simulink model "RiceCooker_harness0"  (R2023b)
settings: Solver=VariableStepAuto  StartTime=0.0  StopTime=5  RelTol=1e-3
settings Model: Creator=20181234  LastModifiedBy=20181234

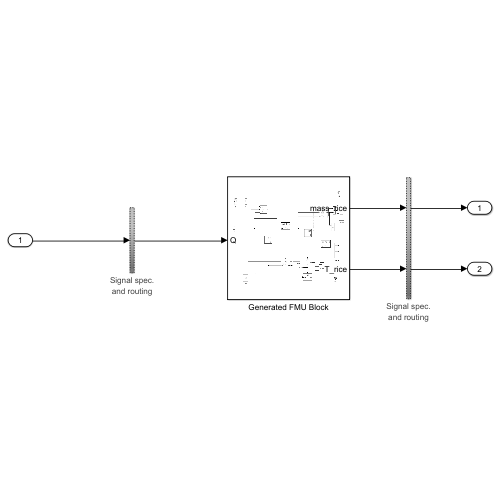
[thumbnail: Simulink's stored preview of the top-level diagram]
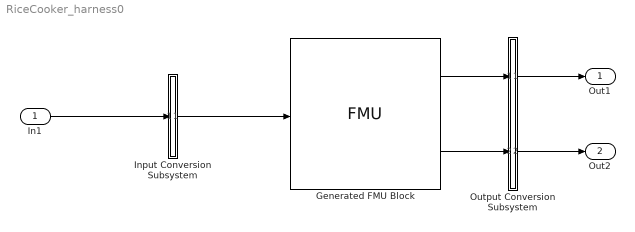
== system RiceCooker_harness0 ==
  In1 : Inport  OutDataTypeStr=double  PortDimensions=[1]  SampleTime=1
  Generated FMU Block : FMU  FMUName=RiceCooker  FMUMode=CoSimulation  FMUSampleTime=1  FMUCreateBusObject=off  FMUInitializeEnumObject=off  T_0=100  m_0=1.5  mask(RiceCooker [Co-Simulation, v2.0]){}
      mask Display:
      | if (exist([Simulink.fileGenControl('get','CacheFolder') '\slprj\_fmu\fd06c610bd597baabc11c1582149db8f\RiceCooker\model.png'],'file'))
      |     image([Simulink.fileGenControl('get','CacheFolder') '\slprj\_fmu\fd06c610bd597baabc11c1582149db8f\RiceCooker\model.png']);
      | else
      |     disp('RiceCooker');
      | end
      | port_label('output',1,'mass_rice');
      | port_label('output',2,'T_rice');
      | port_label('input',1,'Q');
  Input Conversion Subsystem : Subsystem  Tag=__SLT_ICS__  Description=|
      | Signal spec.
      | and routing
      settings: AttributesFormatString=%<Description>
  Output Conversion Subsystem : Subsystem  Tag=__SLT_OCS__  Description=|
      | Signal spec.
      | and routing
      settings: AttributesFormatString=%<Description>
  Out1 : Outport
  Out2 : Outport  Port=2
  wires:
  In1/1 -> Input Conversion Subsystem/1(Inport_1)
  Output Conversion Subsystem/1(Outport_1) -> Out1/1
  Output Conversion Subsystem/2(Outport_2) -> Out2/1
  Input Conversion Subsystem/1(Outport_1) -> Generated FMU Block/1
  Generated FMU Block/1 -> Output Conversion Subsystem/1(Inport_1)
  Generated FMU Block/2 -> Output Conversion Subsystem/2(Inport_2)

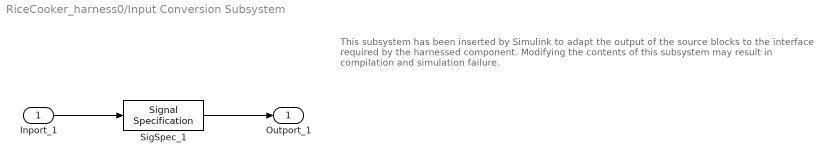
== system RiceCooker_harness0/Input Conversion Subsystem ==
  note: This subsystem has been inserted by Simulink to adapt the output of the source blocks to the interface required by the harnessed component.
      |  Modifying the contents of this subsystem may result in compilation and simulation failure.
  Inport_1 : Inport
  SigSpec_1 : SignalSpecification  OutDataTypeStr=double  Dimensions=[1]  SampleTime=1
  Outport_1 : Outport
  wires:
  SigSpec_1/1 -> Outport_1/1
  Inport_1/1 -> SigSpec_1/1

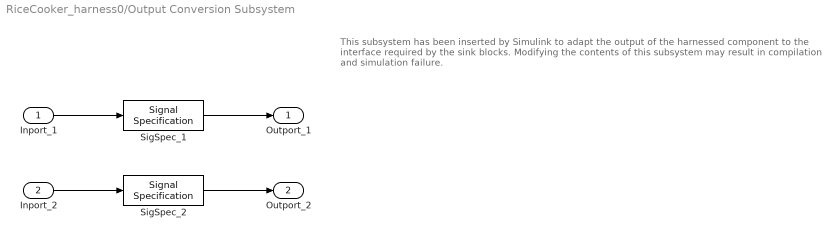
== system RiceCooker_harness0/Output Conversion Subsystem ==
  note: This subsystem has been inserted by Simulink to adapt the output of the harnessed component to the interface required by the sink blocks.
      |  Modifying the contents of this subsystem may result in compilation and simulation failure.
  Inport_1 : Inport
  Inport_2 : Inport  Port=2
  SigSpec_1 : SignalSpecification  OutDataTypeStr=double  Dimensions=[1]  SampleTime=1
  SigSpec_2 : SignalSpecification  OutDataTypeStr=double  Dimensions=[1]  SampleTime=1
  Outport_1 : Outport
  Outport_2 : Outport  Port=2
  wires:
  Inport_1/1 -> SigSpec_1/1
  SigSpec_1/1 -> Outport_1/1
  Inport_2/1 -> SigSpec_2/1
  SigSpec_2/1 -> Outport_2/1
